simulink model "sub_ctof_system"  (R2016b)
settings: Solver=VariableStepAuto  StartTime=0.0  StopTime=10.0  RelTol=1e-3
settings Model: Creator=momen  LastModifiedBy=momen

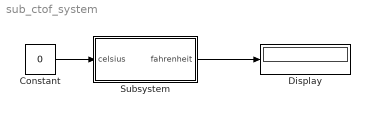
== system sub_ctof_system ==
  Constant : Constant  Value=0
  Display : Display
  Subsystem : Subsystem
  wires:
  Subsystem/1(fahrenheit) -> Display/1
  Constant/1 -> Subsystem/1(celsius)

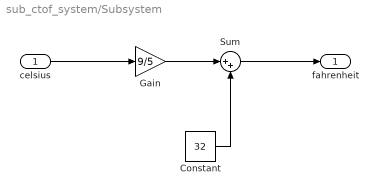
== system sub_ctof_system/Subsystem ==
  celsius : Inport
  Constant : Constant  Value=32
  Gain : Gain  Gain=9/5
  Sum : Sum  Inputs=|++
  fahrenheit : Outport
  wires:
  celsius/1 -> Gain/1
  Gain/1 -> Sum/1
  Constant/1 -> Sum/2
  Sum/1 -> fahrenheit/1
